simulink subsystem "BMSSoCEKF"  (R2024b)
settings: Solver=VariableStepAuto  StartTime=0.0  StopTime=10.0  RelTol=1e-3
undefined symbols (not defined in the file): battery
settings Model: Creator=jjha  LastModifiedBy=jjha
settings OptimizationCC: ReuseModelBlockBuffer=off
settings RTWCC: GPUComputeCapability=3.5

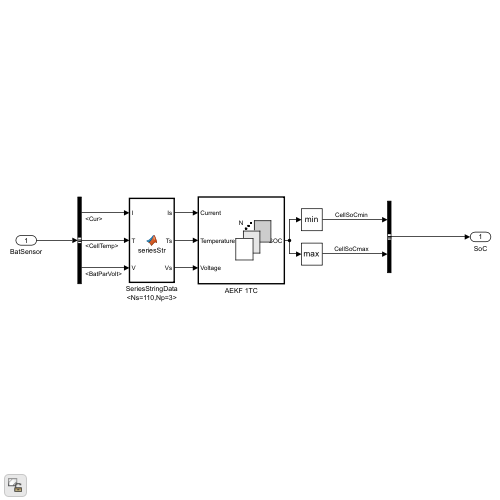
[thumbnail: Simulink's stored preview of the top-level diagram]
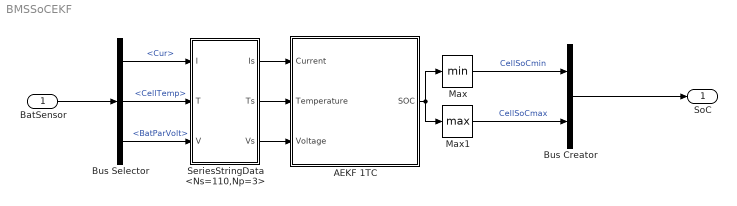
== system BMSSoCEKF ==
  BatSensor : Inport
  AEKF 1TC : Subsystem  TreatAsAtomicUnit=on
  Bus Creator : BusCreator  Inputs=2
  Bus Selector : BusSelector  OutputSignals=Cur,CellTemp,BatParVolt
  Max : MinMax  ZeroCross=off
  Max1 : MinMax  Function=max  ZeroCross=off
  SeriesStringData <Ns=110,Np=3> : MATLAB Function  TreatAsAtomicUnit=on
  SoC : Outport
  wires:
  SeriesStringData <Ns=110,Np=3>/3(Vs) -> AEKF 1TC/3(Voltage)
  SeriesStringData <Ns=110,Np=3>/2(Ts) -> AEKF 1TC/2(Temperature)
  Bus Selector/1 -> SeriesStringData <Ns=110,Np=3>/1(I)  "<Cur>"
  AEKF 1TC/1(SOC) -> Max/1, Max1/1
  Max1/1 -> Bus Creator/2  "CellSoCmax"
  SeriesStringData <Ns=110,Np=3>/1(Is) -> AEKF 1TC/1(Current)
  Bus Selector/2 -> SeriesStringData <Ns=110,Np=3>/2(T)  "<CellTemp>"
  Bus Selector/3 -> SeriesStringData <Ns=110,Np=3>/3(V)  "<BatParVolt>"
  Max/1 -> Bus Creator/1  "CellSoCmin"
  BatSensor/1 -> Bus Selector/1
  Bus Creator/1 -> SoC/1

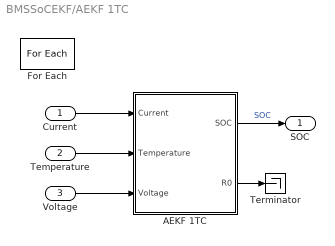
== system BMSSoCEKF/AEKF 1TC ==
  Current : Inport  Partition=on  PartitionDimension=1  PartitionWidth=1  PartitionOffset=0
  Temperature : Inport  Port=2  Partition=on  PartitionDimension=1  PartitionWidth=1  PartitionOffset=0
  Voltage : Inport  Port=3  Partition=on  PartitionDimension=1  PartitionWidth=1  PartitionOffset=0
  AEKF 1TC : Subsystem  mask(Adaptive Extended Kalman Filter SOC estimator){SOC_vec=battery.SOC_vec, T_vec=battery.T_vec, R0_mat=battery.R0_mat, R1_mat=battery.R1_mat, tau1_mat=battery.Tau1_mat, V0_mat=battery.V0_mat, AH_vec=battery.AH_vec, Reol=0.05, Ts=1, Q=1e-8*eye(3), R=1e-2, P0=[1e-5 0 0; 0 1 0; 0 0 0.0125], x0=[battery.iniSOC(1);0;9.4e-3]}
      mask prompts: SOC_vec "Vector of state-of-charge values, SOC"; T_vec "Vector of temperatures, T"; R0_mat "Terminal resistance, R0(SOC,T)"; R1_mat "First polarization resistance, R1(SOC,T)"; tau1_mat "First time constant, tau1(SOC,T)"; V0_mat "No-load voltage, V0(SOC,T)"; AH_vec "Ampere-hour rating, AH(T)"; Reol "End of life resistance"; Ts "Sample time"; Q "Covariance of the process noise, Q"; R "Covariance matrix of the measurement noise, R"; P0 "Initial state error covariance, P0"; x0 "Initial state"
      mask help: This block implements an Adaptive Extended Kalman Filter battery SOC estimator based on a one time constant battery model.
      mask init:
      | C1_mat=tau1_mat./R1_mat;
      | 
      | dV0_mat=zeros(size(V0_mat));
      | [n_soc,m_soc]=size(SOC_vec);
      | if n_soc<m_soc
      |     dV0_mat(2:end,:)=diff(V0_mat,1,1)./diff(SOC_vec');
      | else
      |     dV0_mat(2:end,:)=diff(V0_mat,1,1)./diff(SOC_vec);
      | end
      mask DialogControl Container7 Prompt: System Model
      mask DialogControl Container10 Prompt: Kalman Filter
  For Each : ForEach  DisableCoverage=on
  Terminator : Terminator
  SOC : Outport  ConcatenationDimension=1
  wires:
  AEKF 1TC/2(R0) -> Terminator/1
  Voltage/1 -> AEKF 1TC/3(Voltage)
  Temperature/1 -> AEKF 1TC/2(Temperature)
  AEKF 1TC/1(SOC) -> SOC/1  "SOC"
  Current/1 -> AEKF 1TC/1(Current)

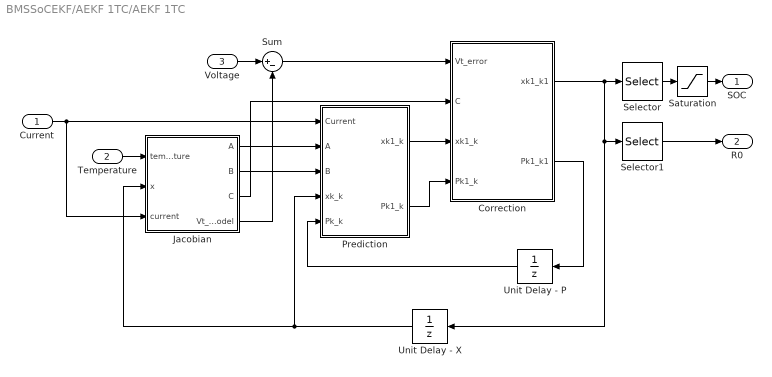
== system BMSSoCEKF/AEKF 1TC/AEKF 1TC ==
  Current : Inport
  Temperature : Inport  Port=2
  Voltage : Inport  Port=3
  Correction : Subsystem
  Jacobian : Subsystem
  Prediction : Subsystem
  Saturation : Saturate  UpperLimit=1  LowerLimit=0
  Selector : Selector  InputPortWidth=3  IndexOptions=Index vector (dialog)  Indices=1  OutputSizes=1
  Selector1 : Selector  InputPortWidth=3  IndexOptions=Index vector (dialog)  Indices=3  OutputSizes=1
  Sum : Sum  Inputs=|+-
  Unit Delay - P : UnitDelay  InitialCondition=P0  SampleTime=Ts  HasFrameUpgradeWarning=on
  Unit Delay - X : UnitDelay  InitialCondition=x0  SampleTime=Ts  HasFrameUpgradeWarning=on
  SOC : Outport  VectorParamsAs1DForOutWhenUnconnected=off
  R0 : Outport  Port=2  VectorParamsAs1DForOutWhenUnconnected=off
  wires:
  Selector1/1 -> R0/1
  Saturation/1 -> SOC/1
  Selector/1 -> Saturation/1
  Current/1 -> Jacobian/3(current), Prediction/1(Current)
  Jacobian/4(Vt_model) -> Sum/2
  Voltage/1 -> Sum/1
  Jacobian/3(C) -> Correction/2(C)
  Jacobian/2(B) -> Prediction/3(B)
  Jacobian/1(A) -> Prediction/2(A)
  Temperature/1 -> Jacobian/1(temperature)
  Sum/1 -> Correction/1(Vt_error)
  Correction/1(xk1_k1) -> Unit Delay - X/1, Selector1/1, Selector/1
  Unit Delay - X/1 -> Prediction/4(xk_k), Jacobian/2(x)
  Unit Delay - P/1 -> Prediction/5(Pk_k)
  Correction/2(Pk1_k1) -> Unit Delay - P/1
  Prediction/2(Pk1_k) -> Correction/4(Pk1_k)
  Prediction/1(xk1_k) -> Correction/3(xk1_k)

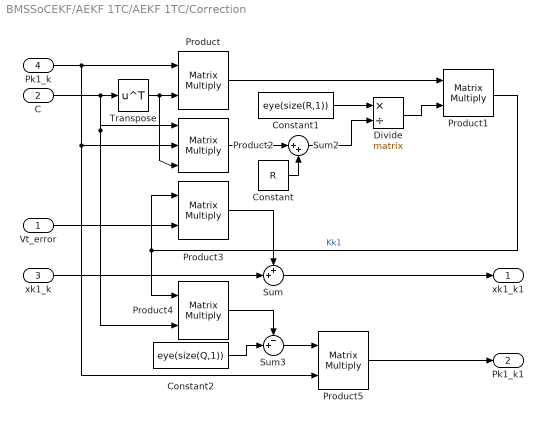
== system BMSSoCEKF/AEKF 1TC/AEKF 1TC/Correction ==
  Vt_error : Inport
  C : Inport  Port=2
  xk1_k : Inport  Port=3
  Pk1_k : Inport  Port=4
  Constant : Constant  Value=R
  Constant1 : Constant  Value=eye(size(R,1))
  Constant2 : Constant  Value=eye(size(Q,1))
  Divide : Product  Inputs=*/  Multiplication=Matrix(*)
  Product{,1,3..5} (5 alike) : Product  Multiplication=Matrix(*)
  Product2 : Product  Inputs=3  Multiplication=Matrix(*)
  Sum : Sum  Inputs=++|
  Sum2 : Sum  Inputs=|++
  Sum3 : Sum  Inputs=-+|
  Transpose : Math  Operator=transpose
  xk1_k1 : Outport
  Pk1_k1 : Outport  Port=2
  wires:
  Product5/1 -> Pk1_k1/1
  Sum3/1 -> Product5/1
  Product4/1 -> Sum3/1
  Constant2/1 -> Sum3/2
  Sum/1 -> xk1_k1/1
  Product3/1 -> Sum/1
  Vt_error/1 -> Product3/2
  xk1_k/1 -> Sum/2
  Constant1/1 -> Divide/1
  Divide/1 -> Product1/2
  Sum2/1 -> Divide/2
  Product1/1 -> Product3/1, Product4/1  "Kk1"
  Constant/1 -> Sum2/2
  Product2/1 -> Sum2/1
  Product/1 -> Product1/1
  Pk1_k/1 -> Product/1, Product2/2, Product5/2
  Transpose/1 -> Product/2, Product2/3
  C/1 -> Transpose/1, Product2/1, Product4/2

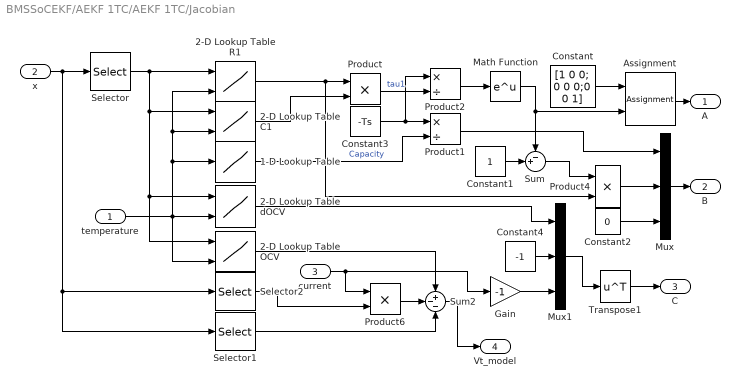
== system BMSSoCEKF/AEKF 1TC/AEKF 1TC/Jacobian ==
  temperature : Inport
  x : Inport  Port=2
  current : Inport  Port=3
  1-D Lookup Table : Lookup_n-D  NumberOfTableDimensions=1  BreakpointsForDimension1=T_vec  Table=AH_vec*3600  InternalRulePriority=Speed  RndMeth=Simplest
  2-D Lookup Table C1 : Lookup_n-D  BreakpointsForDimension1=SOC_vec  BreakpointsForDimension2=T_vec  Table=C1_mat  InternalRulePriority=Speed  RndMeth=Simplest
      settings: InputPortMap=u0,u1
  2-D Lookup Table OCV : Lookup_n-D  BreakpointsForDimension1=SOC_vec  BreakpointsForDimension2=T_vec  Table=V0_mat  InternalRulePriority=Speed  RndMeth=Simplest
      settings: InputPortMap=u0,u1
  2-D Lookup Table R1 : Lookup_n-D  BreakpointsForDimension1=SOC_vec  BreakpointsForDimension2=T_vec  Table=R1_mat  InternalRulePriority=Speed  RndMeth=Simplest
      settings: InputPortMap=u0,u1
  2-D Lookup Table dOCV : Lookup_n-D  BreakpointsForDimension1=SOC_vec  BreakpointsForDimension2=T_vec  Table=dV0_mat  InternalRulePriority=Speed  RndMeth=Simplest
      settings: InputPortMap=u0,u1
  Assignment : Assignment  NumberOfDimensions=2  DiagnosticForDimensions=Warning  IndexOptions=Index vector (dialog),Index vector (dialog)  Indices=2,2  OutputSizes=1,1
  Constant : Constant  Value=|
      | [1 0 0;
      | 0 0 0;0 0 1]
  Constant1 : Constant
  Constant2 : Constant  Value=0
  Constant3 : Constant  Value=-Ts
  Constant4 : Constant  Value=-1
  Gain : Gain  Gain=-1
  Math Function : Math
  Mux : Mux  Inputs=3
  Mux1 : Mux  Inputs=3
  Product : Product
  Product1 : Product  Inputs=*/
  Product2 : Product  Inputs=*/
  Product4 : Product
  Product6 : Product
  Selector : Selector  InputPortWidth=3  IndexOptions=Index vector (dialog)  Indices=1  OutputSizes=1
  Selector1 : Selector  InputPortWidth=3  IndexOptions=Index vector (dialog)  Indices=2  OutputSizes=1
  Selector2 : Selector  InputPortWidth=3  IndexOptions=Index vector (dialog)  Indices=3  OutputSizes=1
  Sum : Sum  Inputs=-+|
  Sum2 : Sum  Inputs=+--
  Transpose1 : Math  Operator=transpose
  A : Outport
  B : Outport  Port=2
  C : Outport  Port=3
  Vt_model : Outport  Port=4
  wires:
  Selector2/1 -> Product6/2
  2-D Lookup Table dOCV/1 -> Mux1/1
  2-D Lookup Table OCV/1 -> Sum2/1
  Sum2/1 -> Vt_model/1
  Transpose1/1 -> C/1
  Mux1/1 -> Transpose1/1
  Selector1/1 -> Sum2/3
  Product6/1 -> Sum2/2
  Constant4/1 -> Mux1/2
  Mux/1 -> B/1
  Product4/1 -> Mux/2
  Product1/1 -> Mux/1
  Sum/1 -> Product4/1
  Constant1/1 -> Sum/2
  Assignment/1 -> A/1
  Product2/1 -> Math Function/1
  Constant3/1 -> Product2/1, Product1/1
  Product/1 -> Product2/2  "tau1"
  2-D Lookup Table C1/1 -> Product/2
  2-D Lookup Table R1/1 -> Product/1, Product4/2
  Math Function/1 -> Assignment/2, Sum/1
  Constant/1 -> Assignment/1
  x/1 -> Selector/1, Selector2/1, Selector1/1
  1-D Lookup Table/1 -> Product1/2  "Capacity"
  Selector/1 -> 2-D Lookup Table R1/1, 2-D Lookup Table C1/1, 2-D Lookup Table dOCV/1, 2-D Lookup Table OCV/1
  temperature/1 -> 2-D Lookup Table OCV/2, 2-D Lookup Table dOCV/2, 1-D Lookup Table/1, 2-D Lookup Table C1/2, 2-D Lookup Table R1/2
  current/1 -> Gain/1, Product6/1
  Gain/1 -> Mux1/3
  Constant2/1 -> Mux/3

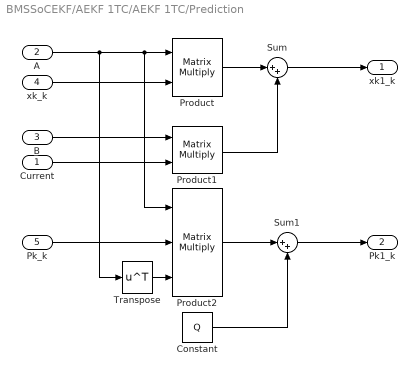
== system BMSSoCEKF/AEKF 1TC/AEKF 1TC/Prediction ==
  Current : Inport
  A : Inport  Port=2
  B : Inport  Port=3
  xk_k : Inport  Port=4
  Pk_k : Inport  Port=5
  Constant : Constant  Value=Q
  Product : Product  Multiplication=Matrix(*)
  Product1 : Product  Multiplication=Matrix(*)
  Product2 : Product  Inputs=3  Multiplication=Matrix(*)
  Sum : Sum  Inputs=|++
  Sum1 : Sum  Inputs=|++
  Transpose : Math  Operator=transpose
  xk1_k : Outport
  Pk1_k : Outport  Port=2
  wires:
  Sum1/1 -> Pk1_k/1
  Constant/1 -> Sum1/2
  Product2/1 -> Sum1/1
  Transpose/1 -> Product2/3
  Pk_k/1 -> Product2/2
  Sum/1 -> xk1_k/1
  Product1/1 -> Sum/2
  Product/1 -> Sum/1
  Current/1 -> Product1/2
  B/1 -> Product1/1
  xk_k/1 -> Product/2
  A/1 -> Product/1, Product2/1, Transpose/1

== matlab function BMSSoCEKF/SeriesStringData <Ns=110,Np=3> ==
  data: I input; Is output; T input; V input; Ts output; Vs output
function [Is,Ts,Vs] = seriesStr(I,T,V)
    Nm=10;
    N=11;
    Np=3;
    Is=zeros(Nm,1);
    Ts=zeros(Nm,1);
    Vs=zeros(Nm,1);
    for itr=1:Nm
        Is(itr,1)=-I/Np;
        Ts(itr,1)=T(itr,1);
        Vs(itr,1)=V(itr,1)/N;
    end
end
